simulink model "rover_arms_learn_1"  (R2021a)
settings: Solver=FixedStepAuto  StartTime=0.0  StopTime=40  FixedStep=0.01  MaxStep=0.4  RelTol=1e-3
undefined symbols (not defined in the file): X, Y, Z
libraries: sm_lib x58, nesl_utility x4, simulink x3
(part 2 of 2)

== matlab function rover_arms_learn_1/MATLAB Function ==
  data: x input; hinge1 output; y input; hinge2 output
function [hinge1, hinge2] = fcn(x,y)

l1 = 39.192
l2 = 39.192

a1=45;
a2=-45;

a1 = deg2rad(a1);
a2 = deg2rad(a2);

Angle = [a1;a2]                 %PRINT
Xd = [x;y]                      %PRINT
%J = [-l2*sin(a1+a2) - l1*sin(a1), -(l2*sin(a1+a2)); l2*cos(a1+a2) + l1*cos(a1), l2*cos(a1+a2)];

for n = 1:10
X  = [cos(a1+a2)*l2 + l1*cos(a1);sin(a1+a2)*l2+l1*sin(a1)];
J = [-l2*sin(a1+a2) - l1*sin(a1), -(l2*sin(a1+a2)); l2*cos(a1+a2) + l1*cos(a1), l2*cos(a1+a2)];
J;
J_inv = inv(J),20;
J_inv;

"hello " ;
n;

Angle = Angle - J_inv*(X-Xd);
a = rad2deg(Angle);

a1 = Angle(1,1);
a2 = Angle(2,1);

end

a = rad2deg(Angle)
hinge1 = a(1,1)
hinge2 = a(2,1)
%rem(a,360)
